simulink model "interpreted_ode"  (R2018b)
settings: Solver=VariableStepAuto  StartTime=0.0  StopTime=30  RelTol=1e-3
settings Model: Creator=kekatos  LastModifiedBy=kekatos

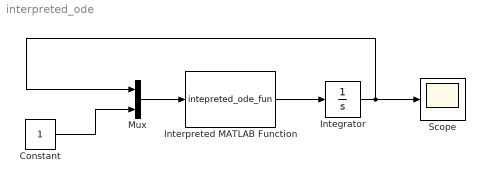
== system interpreted_ode ==
  Constant : Constant
  Integrator : Integrator  InitialCondition=0.5
  Interpreted MATLAB Function : MATLABFcn  MATLABFcn=intepreted_ode_fun  OutputDimensions=2
  Mux : Mux  Inputs=2
  Scope : Scope
  wires:
  Integrator/1 -> Mux/1, Scope/1
  Constant/1 -> Mux/2
  Mux/1 -> Interpreted MATLAB Function/1
  Interpreted MATLAB Function/1 -> Integrator/1
